simulink model "Faulted"  (Simulink 10.3)
settings: Solver=ode23tb  StartTime=0.0  StopTime=2.5  RelTol=1e-3  EnableMultiTasking=on
InitFcn:
  | Ts=20e-6;
libraries: spsDiodeLib x6, spsSeriesRLCBranchLib x4, spsSaturableTransformerLib x3, spsThreePhaseVIMeasurementLib x2, spsThreePhaseProgrammableVoltageSourceLib x1, spsGroundLib x1, spsThreePhaseSeriesRLCBranchLib x1, spspowerguiLib x1
settings Model: Creator=srikanth  LastModifiedBy=Yeaz Mahmud
settings SolverCC: AlgebraicLoopSolver=Auto
settings DataIOCC: LimitDataPoints=on  SaveOutput=off  SaveTime=off
settings DebuggingCC: AlgebraicLoopMsg=none  SolverPrmCheckMsg=warning

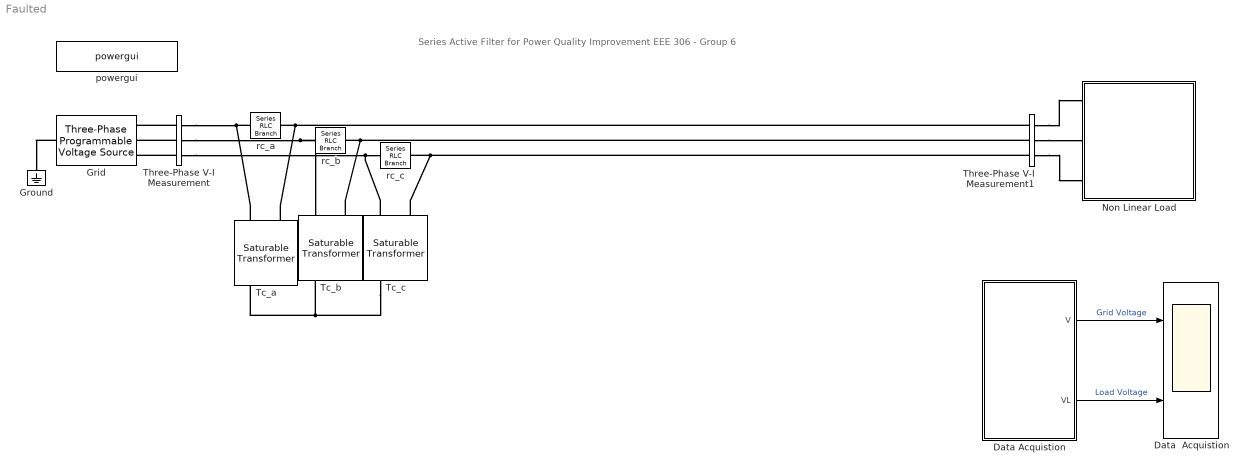
== system Faulted ==
  note: Series Active Filter for Power Quality Improvement
      | EEE 306 - Group 6
  Data  Acquistion : Scope  NumInputPorts=2
  Data Acquistion : Subsystem
      mask Display: fprintf('scopes')
  Grid : spsThreePhaseProgrammableVoltageSourceLib/Three-Phase Programmable Voltage Source  PositiveSequence="[380  0 50]"  VariationEntity=Amplitude  VariationType=Table of time-amplitude pairs  VariationTypeAlt=Step  VariationStep=0.5  VariationRate=10  VariationMagnitude=0.3  VariationFrequency=2  VariationTiming=[1 2]  VariationPhaseA=off  Amplitudes=[1 0.5 1 1.5 1]  TimeValues=[0 0.5 0.7 1.5 1.7]  HarmonicGeneration=on  HarmonicA=[5 0.2 0 2]  HarmonicB=[7 0.05 0 1]  Timing="[0.2  0.4]"  BusType=swing  Pref=0  Qref=0  Qmin=-inf  Qmax=inf
  Ground : spsGroundLib/Ground  LConnTagsString=a
  "Non Linear Load " : Subsystem
      mask Display: fprintf('Non Linear\nLoad')
  Tc_a : spsSaturableTransformerLib/Saturable Transformer  ThreeWindings=off  Hysteresis=off  DataFile='hysteresis.mat'  Measurements=None  UNITS=pu  NominalPower=[4000 50]  Winding1="[380  0.02  0.02 ]"  Winding2="[380  0.02  0.02]"  Winding3="[ 315e3  0.002  0.08 ]"  Saturation=[ 0 0 ;1.016 9.043]*1e-3  CoreLoss=[117 0]  BreakLoop=off  DiscreteSolver=Trapezoidal iterative  DataType=off  InitialFlux=0  TransfoNumber=1
      settings: SourceProductBaseCode=PS
  Tc_b : spsSaturableTransformerLib/Saturable Transformer  ThreeWindings=off  Hysteresis=off  DataFile='hysteresis.mat'  Measurements=None  UNITS=pu  NominalPower=[4000 50]  Winding1="[380  0.02  0.02 ]"  Winding2="[380  0.02  0.02]"  Winding3="[ 315e3  0.002  0.08 ]"  Saturation=[ 0 0 ;1.016 9.043]*1e-3  CoreLoss=[117 0]  BreakLoop=off  DiscreteSolver=Trapezoidal iterative  DataType=off  InitialFlux=0  TransfoNumber=1
      settings: SourceProductBaseCode=PS
  Tc_c : spsSaturableTransformerLib/Saturable Transformer  ThreeWindings=off  Hysteresis=off  DataFile='hysteresis.mat'  Measurements=None  UNITS=pu  NominalPower=[4000 50]  Winding1="[380  0.02  0.02 ]"  Winding2="[380  0.02  0.02]"  Winding3="[ 315e3  0.002  0.08 ]"  Saturation=[ 0 0 ;1.016 9.043]*1e-3  CoreLoss=[117 0]  BreakLoop=off  DiscreteSolver=Trapezoidal iterative  DataType=off  InitialFlux=0  TransfoNumber=1
      settings: SourceProductBaseCode=PS
  Three-Phase V-I Measurement : spsThreePhaseVIMeasurementLib/Three-Phase V-I Measurement  VoltageMeasurement=phase-to-ground  SetLabelV=on  LabelV=Vabc  Vpu=off  VpuLL=off  CurrentMeasurement=yes  SetLabelI=on  LabelI=Iabc  Ipu=off  Pbase=100e6  Vbase=500e3  OutputType=Complex  PhasorSimulation=off  PSBequivalent=0
  Three-Phase V-I Measurement1 : spsThreePhaseVIMeasurementLib/Three-Phase V-I Measurement  VoltageMeasurement=phase-to-ground  SetLabelV=on  LabelV=V_L  Vpu=off  VpuLL=off  CurrentMeasurement=yes  SetLabelI=on  LabelI=I_L  Ipu=off  Pbase=100e6  Vbase=500e3  OutputType=Complex  PhasorSimulation=off  PSBequivalent=0
  powergui : spspowerguiLib/powergui  Priority=1  SimulationMode=Discrete  SampleTime=Ts  frequency=60  Iterations=50  frequencyindice=50  Pbase=100e6  ErrMax=1e-4  UnitsV=kV  UnitsW=MW  buscounter=0  FunctionMessages=off  echomessages=off  EnableUseOfTLC=off  CurrentSourceSwitches=off  DisableSnubberDevices=off  DisableRonSwitches=off  DisableVfSwitches=off  DisplayEquations=off  AutomaticDiscreteSolvers=off  SolverType=Tustin/Backward Euler (TBE)  Interpol=off  ExternalGateDelay=off  methode=off  Ts=0  x0status=blocks  SPID=off  SwTol=0  HookPort=off  NonlinearTolerance=1e-4  nMaxIteration=100  ContinueOnMaxIteration=off  RestoreLinks=warning  ResistiveCurrentMeasurement=off  Frange=[0:2:500]  Ylog=off  Xlog=on  ShowGrid=off  save=off  variable=ZData  structure=voltage_pi  ZoomFFT=off  StartTime=1.5  cycles=10  DisplayStyle=1  fundamental=50  FreqAxis=on  MaxFrequency=1000  frequencyindicesteady=1  RmsSteady=1  display=off
  rc_a : spsSeriesRLCBranchLib/Series RLC Branch  LConnTagsString=__new0  RConnTagsString=__new0  BranchType=RC  Resistance=1  Inductance=1e-3  SetiL0=off  InitialCurrent=0  Capacitance=100e-6  Setx0=off  InitialVoltage=0  Measurements=Branch voltage
  rc_b : spsSeriesRLCBranchLib/Series RLC Branch  LConnTagsString=__new0  RConnTagsString=__new0  BranchType=RC  Resistance=1  Inductance=1e-3  SetiL0=off  InitialCurrent=0  Capacitance=100e-6  Setx0=off  InitialVoltage=0  Measurements=Branch voltage
  rc_c : spsSeriesRLCBranchLib/Series RLC Branch  LConnTagsString=__new0  RConnTagsString=__new0  BranchType=RC  Resistance=1  Inductance=1e-3  SetiL0=off  InitialCurrent=0  Capacitance=100e-6  Setx0=off  InitialVoltage=0  Measurements=Branch voltage
  wires:
  Data Acquistion/1(V) -> Data  Acquistion/1  "Grid Voltage"
  Data Acquistion/2(VL) -> Data  Acquistion/2  "Load Voltage"
  connections:
  Three-Phase V-I Measurement1/LConn2 -- rc_b/LConn1 -- Tc_b/RConn2
  Three-Phase V-I Measurement1/LConn1 -- rc_a/LConn1 -- Tc_a/RConn2
  Grid/LConn1 -- Ground/LConn1
  Three-Phase V-I Measurement/LConn1 -- Grid/RConn1
  Three-Phase V-I Measurement/LConn2 -- Grid/RConn2
  Three-Phase V-I Measurement/LConn3 -- Grid/RConn3
  Three-Phase V-I Measurement1/RConn2 -- "Non Linear Load "/LConn2
  Three-Phase V-I Measurement1/LConn3 -- rc_c/LConn1 -- Tc_c/RConn2
  rc_a/RConn1 -- Three-Phase V-I Measurement/RConn1 -- Tc_a/RConn1
  rc_b/RConn1 -- Three-Phase V-I Measurement/RConn2 -- Tc_b/RConn1
  rc_c/RConn1 -- Three-Phase V-I Measurement/RConn3 -- Tc_c/RConn1
  Three-Phase V-I Measurement1/RConn3 -- "Non Linear Load "/LConn3
  Three-Phase V-I Measurement1/RConn1 -- "Non Linear Load "/LConn1
  Tc_c/LConn1 -- Tc_a/LConn1 -- Tc_b/LConn1

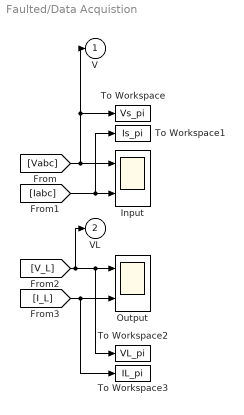
== system Faulted/Data Acquistion ==
  Input : Scope  NumInputPorts=2
  Output : Scope  NumInputPorts=2
  To Workspace : ToWorkspace  VariableName=Vs_pi  SampleTime=Ts
  To Workspace1 : ToWorkspace  VariableName=Is_pi  SampleTime=Ts
  To Workspace2 : ToWorkspace  VariableName=VL_pi  SampleTime=Ts
  To Workspace3 : ToWorkspace  VariableName=IL_pi  SampleTime=Ts
  V : Outport
  VL : Outport  Port=2
  wires:
  [Vabc] -> Input/1, V/1, To Workspace/1
  [Iabc] -> Input/2, To Workspace1/1
  [V_L] -> VL/1, Output/1, To Workspace2/1
  [I_L] -> Output/2, To Workspace3/1

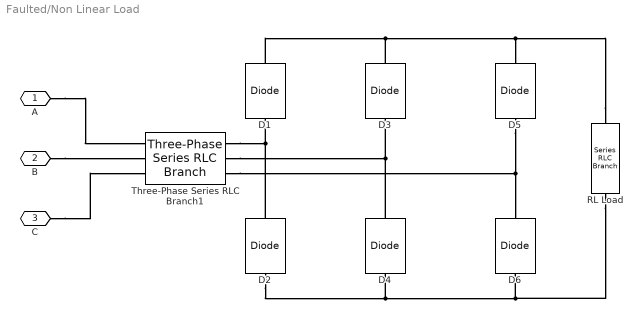
== system Faulted/Non Linear Load  ==
  D{1..6} (6 alike) : spsDiodeLib/Diode  Ron=0.001  Lon=0  Vf=0.8  IC=0  UseSnubber=off  Rs=500  Cs=250e-9  Measurements=off
  RL Load : spsSeriesRLCBranchLib/Series RLC Branch  LConnTagsString=__new0  RConnTagsString=__new0  BranchType=RL  Resistance=60  Inductance=0.15e-3  SetiL0=off  InitialCurrent=0  Capacitance=1e-6  Setx0=off  InitialVoltage=0  Measurements=None
  Three-Phase Series RLC Branch1 : spsThreePhaseSeriesRLCBranchLib/Three-Phase Series RLC Branch  LConnTagsString=A|B|C  RConnTagsString=A|B|C  BranchType=RL  Resistance=0.4  Inductance=15e-3  Capacitance=1e-6  Measurements=None
  A : PMIOPort  Side=Left
  B : PMIOPort  Port=2  Side=Left
  C : PMIOPort  Port=3  Side=Left
  connections:
  C/RConn1 -- Three-Phase Series RLC Branch1/LConn3
  B/RConn1 -- Three-Phase Series RLC Branch1/LConn2
  A/RConn1 -- Three-Phase Series RLC Branch1/LConn1
  Three-Phase Series RLC Branch1/RConn3 -- D6/RConn1 -- D5/LConn1
  Three-Phase Series RLC Branch1/RConn2 -- D4/RConn1 -- D3/LConn1
  RL Load/RConn1 -- D6/LConn1 -- D4/LConn1 -- D2/LConn1
  RL Load/LConn1 -- D5/RConn1 -- D3/RConn1 -- D1/RConn1
  Three-Phase Series RLC Branch1/RConn1 -- D2/RConn1 -- D1/LConn1
